simulink model "test_SwitchSensor"  (R2021b)
settings: Solver=FixedStepAuto  StartTime=0.0  StopTime=10.0  FixedStep=Ts  RelTol=1e-3
libraries: LiftMotionControlLibrary x1
settings Model: Creator=manue  LastModifiedBy=manue
settings DataIOCC: SaveFormat=StructureWithTime

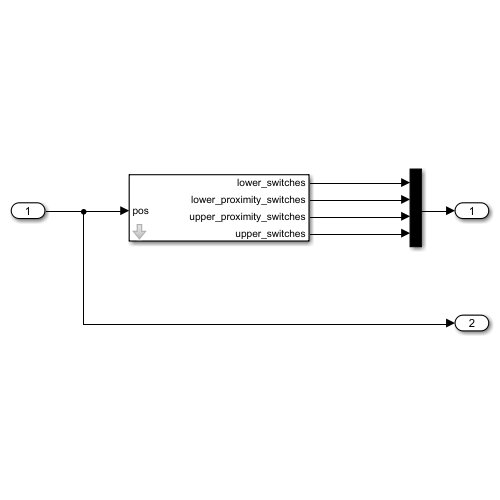
[thumbnail: Simulink's stored preview of the top-level diagram]
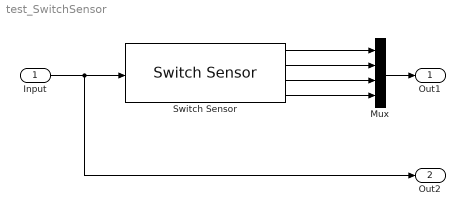
== system test_SwitchSensor ==
  Input : Inport
  Mux : Mux
  Switch Sensor : LiftMotionControlLibrary/Switch Sensor  lower_proximity_sensor_positions=lower_proximity_sensor_positions  upper_proximity_sensor_positions=upper_proximity_sensor_positions  lower_floor_sensor_positions=lower_floor_sensor_positions  upper_floor_sensor_positions=upper_floor_sensor_positions  num_floors=num_floors  sensor_height=sensor_height
  Out1 : Outport
  Out2 : Outport  Port=2
  wires:
  Input/1 -> Out2/1, Switch Sensor/1
  Switch Sensor/1 -> Mux/1
  Switch Sensor/2 -> Mux/2
  Switch Sensor/3 -> Mux/3
  Switch Sensor/4 -> Mux/4
  Mux/1 -> Out1/1
